simulink model "dsf_ut"  (Simulink 8.1)
settings: Solver=FixedStepDiscrete  StartTime=0.0  StopTime=Inf  FixedStep=0.005  RelTol=1e-3
libraries: siltestlib x8, dsf x1
settings Model: Creator=xsellart  LastModifiedBy=AT015555
settings DataIOCC: SignalLoggingSaveFormat=Dataset
settings OptimizationCC: ExpressionDepthLimit=128
settings DebuggingCC: FcnCallInpInsideContextMsg=EnableAllAsError
settings GRTTargetCC: CombineOutputUpdateFcns=on  GRTInterface=off

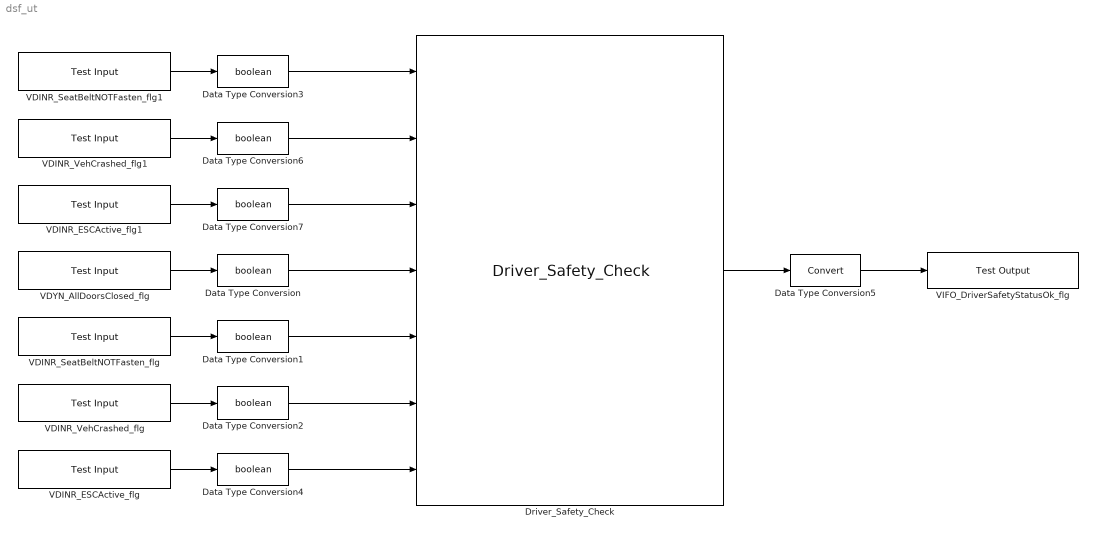
== system dsf_ut ==
  Data Type Conversion{,1..4,6..7} (7 alike) : DataTypeConversion  OutDataTypeStr=boolean
  Data Type Conversion5 : DataTypeConversion
  Driver_Safety_Check : dsf/Driver_Safety_Check
  VDINR_ESCActive_flg : siltestlib/Test Input  varname=VDINR_TCSActive_flg  sampletime=0.005
  VDINR_ESCActive_flg1 : siltestlib/Test Input  varname=VDINR_LRDoorOpen_flg  sampletime=0.005
  VDINR_SeatBeltNOTFasten_flg : siltestlib/Test Input  varname=VDINR_SeatBeltNOTFasten_flg  sampletime=0.005
  VDINR_SeatBeltNOTFasten_flg1 : siltestlib/Test Input  varname=VDINR_DriverDoorOpen_flg  sampletime=0.005
  VDINR_VehCrashed_flg : siltestlib/Test Input  varname=VDINR_VehCrashed_flg  sampletime=0.005
  VDINR_VehCrashed_flg1 : siltestlib/Test Input  varname=VDINR_PassengerDoorOpen_flg  sampletime=0.005
  "VDYN_AllDoorsClosed_flg " : siltestlib/Test Input  varname=VDINR_RRDoorOpen_flg  sampletime=0.005
  "VIFO_DriverSafetyStatusOk_flg " : siltestlib/Test Output  varname=VIFO_DriverSafetyStatusOk_flg  sampletime=-1
  wires:
  "VDYN_AllDoorsClosed_flg "/1 -> Data Type Conversion/1
  Data Type Conversion3/1 -> Driver_Safety_Check/1
  VDINR_SeatBeltNOTFasten_flg/1 -> Data Type Conversion1/1
  VDINR_VehCrashed_flg/1 -> Data Type Conversion2/1
  VDINR_ESCActive_flg/1 -> Data Type Conversion4/1
  Data Type Conversion6/1 -> Driver_Safety_Check/2
  Data Type Conversion7/1 -> Driver_Safety_Check/3
  Data Type Conversion/1 -> Driver_Safety_Check/4
  Driver_Safety_Check/1 -> Data Type Conversion5/1
  Data Type Conversion5/1 -> "VIFO_DriverSafetyStatusOk_flg "/1
  Data Type Conversion1/1 -> Driver_Safety_Check/5
  Data Type Conversion2/1 -> Driver_Safety_Check/6
  Data Type Conversion4/1 -> Driver_Safety_Check/7
  VDINR_SeatBeltNOTFasten_flg1/1 -> Data Type Conversion3/1
  VDINR_VehCrashed_flg1/1 -> Data Type Conversion6/1
  VDINR_ESCActive_flg1/1 -> Data Type Conversion7/1
